simulink model "sampleModel26"  (Simulink 9.1)
settings: Solver=VariableStepAuto  StartTime=0.0  StopTime=10.0  RelTol=1e-3
undefined symbols (not defined in the file): DiscIntNeverNeededParam, Newton, Raphson
libraries: simulink x50
(part 2 of 2)

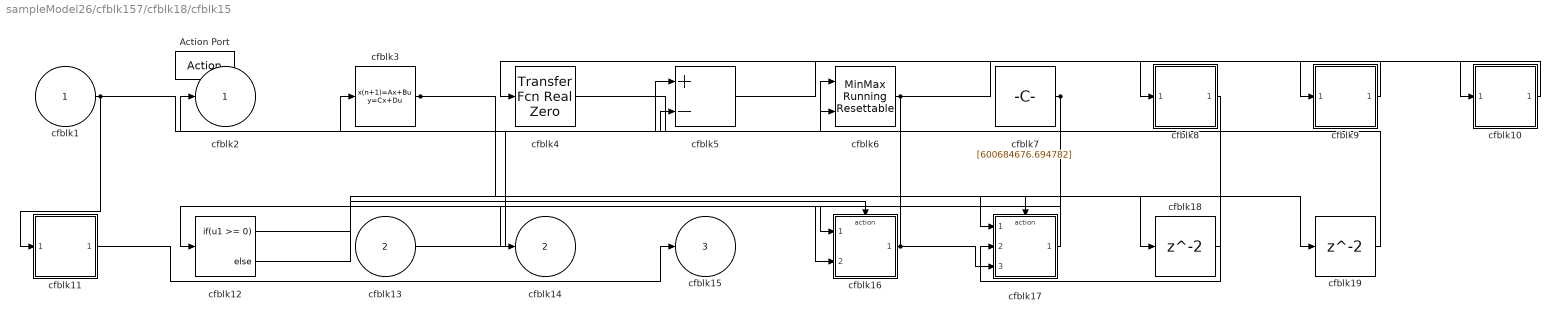
== system sampleModel26/cfblk157/cfblk18/cfblk15 ==
  cfblk1 : Inport
  cfblk13 : Inport  Port=2
  Action Port : ActionPort  ActionType=else
  cfblk10 : Subsystem
  cfblk11 : Subsystem
  cfblk12 : If  IfExpression=u1 >= 0  SampleTime=1
  cfblk16 : Subsystem  TreatAsAtomicUnit=on
  cfblk17 : Subsystem  TreatAsAtomicUnit=on
  cfblk18 : Delay
  cfblk19 : Delay
  cfblk3 : DiscreteStateSpace  SampleTime=-1
  cfblk4 : simulink/Discrete/Transfer Fcn Real Zero  ZeroZ=0.75  ICPrevInput=0.0  DoSatur=off
      settings: SourceProductName=Simulink  SourceProductBaseCode=SL
  cfblk5 : Sum  Inputs=+-
  cfblk6 : simulink/Math Operations/MinMax Running Resettable  Function=min  vinit=0.0
  cfblk7 : Constant  Value=[600684676.694782]  SampleTime=1
  cfblk8 : Subsystem
  cfblk9 : Subsystem
  cfblk2 : Outport
  cfblk14 : Outport  Port=2
  cfblk15 : Outport  Port=3
  wires:
  cfblk10/1(cfblk2) -> cfblk4/1
  cfblk3/1 -> cfblk18/1, cfblk19/1
  cfblk13/1 -> cfblk6/1
  cfblk1/1 -> cfblk11/1(cfblk1), cfblk5/2
  cfblk6/1 -> cfblk12/1, cfblk9/1(cfblk1)
  cfblk4/1 -> cfblk6/2
  cfblk5/1 -> cfblk10/1(cfblk1)
  cfblk11/1(cfblk2) -> cfblk15/1
  cfblk8/1(cfblk2) -> cfblk17/2(cfblk7)
  cfblk7/1 -> cfblk16/1(cfblk1), cfblk16/2(cfblk10), cfblk14/1
  cfblk17/1(cfblk2) -> cfblk2/1
  cfblk9/1(cfblk2) -> cfblk8/1(cfblk1)
  cfblk16/1(cfblk2) -> cfblk17/3(cfblk8), cfblk3/1
  cfblk12/1 -> cfblk16/Action
  cfblk12/2 -> cfblk17/Action
  cfblk18/1 -> cfblk17/1(cfblk1)
  cfblk19/1 -> cfblk5/1

== system sampleModel26/cfblk157/cfblk18/cfblk5 ==
  cfblk1 : Inport
  cfblk2 : Outport
  wires:
  cfblk1/1 -> cfblk2/1

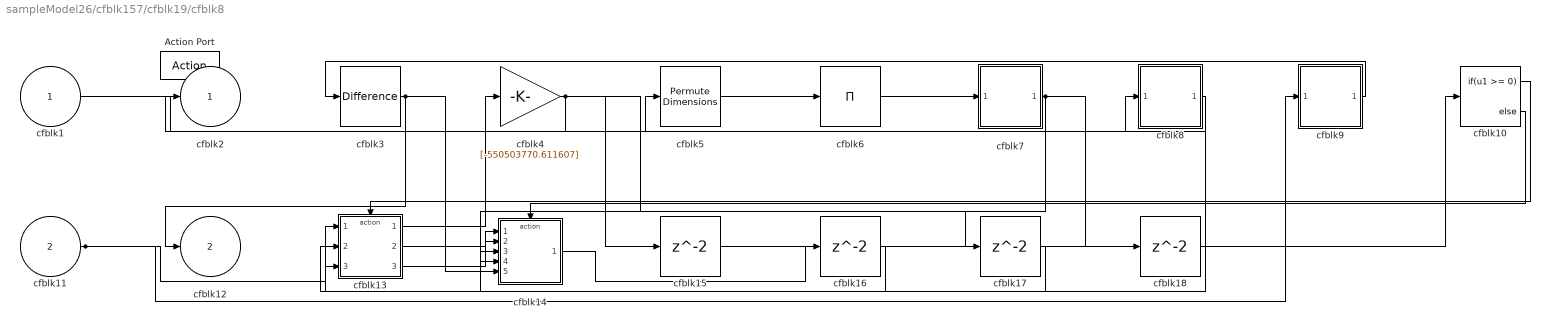
== system sampleModel26/cfblk157/cfblk19/cfblk8 ==
  cfblk1 : Inport
  cfblk11 : Inport  Port=2
  Action Port : ActionPort  ActionType=then
  cfblk10 : If  IfExpression=u1 >= 0  SampleTime=1
  cfblk13 : Subsystem  TreatAsAtomicUnit=on
  cfblk14 : Subsystem  TreatAsAtomicUnit=on
  cfblk{15..18} (4 alike) : Delay
  cfblk3 : simulink/Discrete/Difference  ICPrevInput=0.0  OutMin=[]  OutMax=[]  OutDataTypeStr=Inherit: Inherit via back propagation  OutDataType=fixdt(1, 16)  OutScaling=2^-10  DoSatur=off
  cfblk4 : Gain  Gain=[-550503770.611607]
  cfblk5 : PermuteDimensions
  cfblk6 : Product  Inputs=*
  cfblk7 : Subsystem
  cfblk8 : Subsystem
  cfblk9 : Subsystem
  cfblk2 : Outport
  cfblk12 : Outport  Port=2
  wires:
  cfblk6/1 -> cfblk7/1(cfblk1)
  cfblk1/1 -> cfblk8/1(cfblk1)
  cfblk5/1 -> cfblk6/1
  cfblk9/1(cfblk2) -> cfblk3/1
  cfblk3/1 -> cfblk12/1, cfblk14/5(cfblk17)
  cfblk13/1(cfblk2) -> cfblk4/1
  cfblk4/1 -> cfblk2/1, cfblk15/1, cfblk17/1
  cfblk7/1(cfblk2) -> cfblk14/4(cfblk16), cfblk18/1
  cfblk8/1(cfblk2) -> cfblk13/1(cfblk1)
  cfblk11/1 -> cfblk9/1(cfblk1), cfblk13/3(cfblk14)
  cfblk13/2(cfblk15) -> cfblk14/1(cfblk1)
  cfblk13/3(cfblk16) -> cfblk14/2(cfblk14)
  cfblk10/1 -> cfblk13/Action
  cfblk10/2 -> cfblk14/Action
  cfblk15/1 -> cfblk10/1
  cfblk14/1(cfblk2) -> cfblk16/1
  cfblk16/1 -> cfblk13/2(cfblk13)
  cfblk17/1 -> cfblk14/3(cfblk15)
  cfblk18/1 -> cfblk5/1

== system sampleModel26/cfblk157/cfblk19/cfblk9 ==
  cfblk1 : Inport
  cfblk14 : Inport  Port=2
  cfblk15 : Inport  Port=3
  Action Port : ActionPort  ActionType=else
  cfblk10 : Subsystem
  cfblk11 : Subsystem
  cfblk12 : Subsystem
  cfblk13 : Subsystem
  cfblk3 : simulink/Continuous/PID Controller (2DOF)  Controller=PID  TimeDomain=Discrete-time  SampleTime=-1  IntegratorMethod=Forward Euler  FilterMethod=Forward Euler  Form=Parallel  UseFilter=on  ControllerParametersSource=internal  P=1  I=1  D=0  N=100  b=1  c=1  InitialConditionSource=internal  InitialConditionForIntegrator=0  InitialConditionForFilter=0  ExternalReset=none  LimitOutput=off  UpperSaturationLimit=inf  LowerSaturationLimit=-inf  LinearizeAsGain=off  AntiWindupMode=none  Kb=1  TrackingMode=off  Kt=1  PParamMin=[]  PParamMax=[]  IParamMin=[]  IParamMax=[]  DParamMin=[]  DParamMax=[]  NParamMin=[]  NParamMax=[]  bParamMin=[]  bParamMax=[]  cParamMin=[]  cParamMax=[]  KbParamMin=[]  KbParamMax=[]  KtParamMin=[]  KtParamMax=[]  POutMin=[]  POutMax=[]  IOutMin=[]  IOutMax=[]  DOutMin=[]  DOutMax=[]  NOutMin=[]  NOutMax=[]  bOutMin=[]  bOutMax=[]  cOutMin=[]  cOutMax=[]  KbOutMin=[]  KbOutMax=[]  KtOutMin=[]  KtOutMax=[]  IntegratorOutMin=[]  IntegratorOutMax=[]  FilterOutMin=[]  FilterOutMax=[]  SumOutMin=[]  SumOutMax=[]  Sum1OutMin=[]  Sum1OutMax=[]  Sum2OutMin=[]  Sum2OutMax=[]  Sum3OutMin=[]  Sum3OutMax=[]  SumI1OutMin=[]  SumI1OutMax=[]  SumI2OutMin=[]  SumI2OutMax=[]  SumI3OutMin=[]  SumI3OutMax=[]  SumDOutMin=[]  SumDOutMax=[]  SaturationOutMin=[]  SaturationOutMax=[]  IntegratorContinuousStateAttributes=''  IntegratorStateMustResolveToSignalObject=off  IntegratorRTWStateStorageClass=Auto  FilterContinuousStateAttributes=''  FilterStateMustResolveToSignalObject=off  FilterRTWStateStorageClass=Auto  DifferentiatorICPrevScaledInput=0  DifferentiatorOutMin=[]  DifferentiatorOutMax=[]  FilterDiffOutCoefMin=[]  FilterDiffOutCoefMax=[]  SumDenOutMin=[]  SumDenOutMax=[]  SumNumOutMin=[]  SumNumOutMax=[]  ReciprocalOutMin=[]  ReciprocalOutMax=[]  DivideOutMin=[]  DivideOutMax=[]  TunerSelectOption=Transfer Function Based (PID Tuner App)
  cfblk4 : Sin  TimeSource=Use external signal  SampleTime=0
  cfblk5 : Sqrt  Operator=rSqrt  AlgorithmType=Newton-Raphson  SaturateOnIntegerOverflow=on
  cfblk6 : Sum  Inputs=-+
  cfblk7 : Constant  Value=[532303264.027651]  SampleTime=1
  cfblk8 : Constant  Value=[583399414.909313]  SampleTime=1
  cfblk9 : Subsystem
  cfblk2 : Outport
  cfblk16 : Outport  Port=2
  wires:
  cfblk6/1 -> cfblk10/1(cfblk1)
  cfblk11/1(cfblk2) -> cfblk4/1
  cfblk3/1 -> cfblk9/1(cfblk1)
  cfblk12/1(cfblk2) -> cfblk2/1
  cfblk13/1(cfblk2) -> cfblk5/1
  cfblk10/1(cfblk2) -> cfblk12/1(cfblk1)
  cfblk8/1 -> cfblk13/1(cfblk1)
  cfblk5/1 -> cfblk6/1
  cfblk9/1(cfblk2) -> cfblk16/1
  cfblk7/1 -> cfblk3/1
  cfblk4/1 -> cfblk6/2
  cfblk14/1 -> cfblk3/2
  cfblk15/1 -> cfblk11/1(cfblk1)

== system sampleModel26/cfblk160/cfblk17/cfblk11 ==
  cfblk1 : Inport
  cfblk2 : Outport
  wires:
  cfblk1/1 -> cfblk2/1

== system sampleModel26/cfblk160/cfblk18/cfblk6 ==
  cfblk1 : Inport
  cfblk2 : Outport
  wires:
  cfblk1/1 -> cfblk2/1

== system sampleModel26/cfblk160/cfblk18/cfblk7 ==
  cfblk1 : Inport
  cfblk2 : Outport
  wires:
  cfblk1/1 -> cfblk2/1

== system sampleModel26/cfblk160/cfblk18/cfblk8 ==
  cfblk1 : Inport
  cfblk2 : Outport
  wires:
  cfblk1/1 -> cfblk2/1

== system sampleModel26/cfblk160/cfblk18/cfblk9 ==
  cfblk1 : Inport
  cfblk2 : Outport
  wires:
  cfblk1/1 -> cfblk2/1

== system sampleModel26/cfblk157/cfblk18/cfblk12/cfblk13 ==
  cfblk1 : Inport
  cfblk12 : Inport  Port=2
  cfblk13 : Inport  Port=3
  Action Port : ActionPort  ActionType=then
  cfblk10 : Sum  Inputs=+-
  cfblk11 : Constant  Value=[603434454.897052]  SampleTime=1
  cfblk3 : DiscreteFir
  cfblk4 : DiscreteTransferFcn
  cfblk5 : DiscreteTransferFcn
  cfblk6 : Delay
  cfblk7 : simulink/Discrete/Transfer Fcn First Order  PoleZ=0.95  ICPrevOutput=0.0  DoSatur=off
      settings: SourceProductName=Simulink
  cfblk8 : Rounding
  cfblk9 : PermuteDimensions
  cfblk2 : Outport
  wires:
  cfblk6/1 -> cfblk8/1
  cfblk12/1 -> cfblk7/1
  cfblk1/1 -> cfblk2/1
  cfblk11/1 -> cfblk9/1
  cfblk9/1 -> cfblk4/1
  cfblk4/1 -> cfblk6/1
  cfblk7/1 -> cfblk5/1
  cfblk13/1 -> cfblk3/1
  cfblk3/1 -> cfblk10/1
  cfblk5/1 -> cfblk10/2

== system sampleModel26/cfblk157/cfblk18/cfblk12/cfblk14 ==
  cfblk1 : Inport
  cfblk14 : Inport  Port=2
  cfblk15 : Inport  Port=3
  Action Port : ActionPort  ActionType=else
  cfblk10 : Sum  Inputs=|++
  cfblk11 : Sum  Inputs=+-
  cfblk12 : simulink/Math Operations/Slider Gain  gain=1  low=0  high=2
  cfblk13 : Constant  Value=[170798699.836633]  SampleTime=1
  cfblk3 : simulink/Discrete/Transfer Fcn First Order  PoleZ=0.95  ICPrevOutput=0.0  DoSatur=off
      settings: SourceProductName=Simulink
  cfblk4 : DiscreteZeroPole  Poles=[0 0.5]  Gain=1  SampleTime=-1
  cfblk5 : Delay
  cfblk6 : DiscreteTransferFcn
  cfblk7 : Sqrt  Operator=rSqrt  AlgorithmType=Newton-Raphson  SaturateOnIntegerOverflow=on
  cfblk8 : Polyval  Coefs=[ +2.081618890e-019, -1.441693666e-014, +4.719686976e-010, -8.536869453e-006, +1.621573104e-001, -8.087801117e+001 ]
  cfblk9 : Sin  TimeSource=Use external signal  SampleTime=0
  cfblk2 : Outport
  cfblk16 : Outport  Port=2
  wires:
  cfblk5/1 -> cfblk4/1
  cfblk14/1 -> cfblk10/1
  cfblk13/1 -> cfblk5/1
  cfblk10/1 -> cfblk3/1
  cfblk11/1 -> cfblk16/1
  cfblk7/1 -> cfblk9/1
  cfblk8/1 -> cfblk2/1
  cfblk4/1 -> cfblk7/1
  cfblk6/1 -> cfblk11/1
  cfblk1/1 -> cfblk12/1
  cfblk9/1 -> cfblk11/2
  cfblk12/1 -> cfblk10/2
  cfblk15/1 -> cfblk6/1
  cfblk3/1 -> cfblk8/1

== system sampleModel26/cfblk157/cfblk18/cfblk12/cfblk9 ==
  cfblk1 : Inport
  cfblk2 : Outport
  wires:
  cfblk1/1 -> cfblk2/1

== system sampleModel26/cfblk157/cfblk18/cfblk13/cfblk8 ==
  cfblk1 : Inport
  cfblk2 : Outport
  wires:
  cfblk1/1 -> cfblk2/1

== system sampleModel26/cfblk157/cfblk18/cfblk14/cfblk4 ==
  cfblk1 : Inport
  cfblk2 : Outport
  wires:
  cfblk1/1 -> cfblk2/1

== system sampleModel26/cfblk157/cfblk18/cfblk14/cfblk5 ==
  cfblk1 : Inport
  cfblk2 : Outport
  wires:
  cfblk1/1 -> cfblk2/1

== system sampleModel26/cfblk157/cfblk18/cfblk14/cfblk6 ==
  cfblk1 : Inport
  cfblk2 : Outport
  wires:
  cfblk1/1 -> cfblk2/1

== system sampleModel26/cfblk157/cfblk18/cfblk15/cfblk10 ==
  cfblk1 : Inport
  cfblk2 : Outport
  wires:
  cfblk1/1 -> cfblk2/1

== system sampleModel26/cfblk157/cfblk18/cfblk15/cfblk11 ==
  cfblk1 : Inport
  cfblk2 : Outport
  wires:
  cfblk1/1 -> cfblk2/1

== system sampleModel26/cfblk157/cfblk18/cfblk15/cfblk16 ==
  cfblk1 : Inport
  cfblk10 : Inport  Port=2
  Action Port : ActionPort  ActionType=then
  cfblk11 : Delay
  cfblk12 : Delay
  cfblk3 : UnitDelay  SampleTime=-1
  cfblk4 : simulink/Continuous/PID Controller (2DOF)  Controller=PID  TimeDomain=Discrete-time  SampleTime=-1  IntegratorMethod=Forward Euler  FilterMethod=Forward Euler  Form=Parallel  UseFilter=on  ControllerParametersSource=internal  P=1  I=1  D=0  N=100  b=1  c=1  InitialConditionSource=internal  InitialConditionForIntegrator=0  InitialConditionForFilter=0  ExternalReset=none  LimitOutput=off  UpperSaturationLimit=inf  LowerSaturationLimit=-inf  LinearizeAsGain=off  AntiWindupMode=none  Kb=1  TrackingMode=off  Kt=1  PParamMin=[]  PParamMax=[]  IParamMin=[]  IParamMax=[]  DParamMin=[]  DParamMax=[]  NParamMin=[]  NParamMax=[]  bParamMin=[]  bParamMax=[]  cParamMin=[]  cParamMax=[]  KbParamMin=[]  KbParamMax=[]  KtParamMin=[]  KtParamMax=[]  POutMin=[]  POutMax=[]  IOutMin=[]  IOutMax=[]  DOutMin=[]  DOutMax=[]  NOutMin=[]  NOutMax=[]  bOutMin=[]  bOutMax=[]  cOutMin=[]  cOutMax=[]  KbOutMin=[]  KbOutMax=[]  KtOutMin=[]  KtOutMax=[]  IntegratorOutMin=[]  IntegratorOutMax=[]  FilterOutMin=[]  FilterOutMax=[]  SumOutMin=[]  SumOutMax=[]  Sum1OutMin=[]  Sum1OutMax=[]  Sum2OutMin=[]  Sum2OutMax=[]  Sum3OutMin=[]  Sum3OutMax=[]  SumI1OutMin=[]  SumI1OutMax=[]  SumI2OutMin=[]  SumI2OutMax=[]  SumI3OutMin=[]  SumI3OutMax=[]  SumDOutMin=[]  SumDOutMax=[]  SaturationOutMin=[]  SaturationOutMax=[]  IntegratorContinuousStateAttributes=''  IntegratorStateMustResolveToSignalObject=off  IntegratorRTWStateStorageClass=Auto  FilterContinuousStateAttributes=''  FilterStateMustResolveToSignalObject=off  FilterRTWStateStorageClass=Auto  DifferentiatorICPrevScaledInput=0  DifferentiatorOutMin=[]  DifferentiatorOutMax=[]  FilterDiffOutCoefMin=[]  FilterDiffOutCoefMax=[]  SumDenOutMin=[]  SumDenOutMax=[]  SumNumOutMin=[]  SumNumOutMax=[]  ReciprocalOutMin=[]  ReciprocalOutMax=[]  DivideOutMin=[]  DivideOutMax=[]  TunerSelectOption=Transfer Function Based (PID Tuner App)
  cfblk5 : Sqrt  SaturateOnIntegerOverflow=on
  cfblk6 : simulink/Math Operations/MinMax Running Resettable  Function=min  vinit=0.0
  cfblk7 : ComplexToRealImag
  cfblk8 : Sum  Inputs=+
  cfblk9 : Constant  Value=[-275406093.401909]  SampleTime=1
  cfblk2 : Outport
  wires:
  cfblk6/1 -> cfblk5/1
  cfblk4/1 -> cfblk8/1
  cfblk5/1 -> cfblk3/1
  cfblk3/1 -> cfblk7/1
  cfblk10/1 -> cfblk2/1
  cfblk1/1 -> cfblk4/2
  cfblk8/1 -> cfblk6/2
  cfblk7/1 -> cfblk11/1
  cfblk11/1 -> cfblk4/1
  cfblk7/2 -> cfblk12/1
  cfblk12/1 -> cfblk6/1

== system sampleModel26/cfblk157/cfblk18/cfblk15/cfblk17 ==
  cfblk1 : Inport
  cfblk7 : Inport  Port=2
  cfblk8 : Inport  Port=3
  Action Port : ActionPort  ActionType=else
  cfblk3 : Reshape
  cfblk4 : Product  Inputs=**
  cfblk5 : PermuteDimensions
  cfblk6 : ComplexToRealImag
  cfblk2 : Outport
  wires:
  cfblk6/1 -> cfblk2/1
  cfblk1/1 -> cfblk5/1
  cfblk8/1 -> cfblk3/1
  cfblk6/2 -> cfblk4/1
  cfblk5/1 -> cfblk4/2
  cfblk3/1 -> cfblk6/1

== system sampleModel26/cfblk157/cfblk18/cfblk15/cfblk8 ==
  cfblk1 : Inport
  cfblk2 : Outport
  wires:
  cfblk1/1 -> cfblk2/1

== system sampleModel26/cfblk157/cfblk18/cfblk15/cfblk9 ==
  cfblk1 : Inport
  cfblk2 : Outport
  wires:
  cfblk1/1 -> cfblk2/1

== system sampleModel26/cfblk157/cfblk19/cfblk8/cfblk13 ==
  cfblk1 : Inport
  cfblk13 : Inport  Port=2
  cfblk14 : Inport  Port=3
  Action Port : ActionPort  ActionType=then
  cfblk10 : MinMax  Function=max  Inputs=3
  cfblk11 : Constant  Value=[-226330828.269443]  SampleTime=1
  cfblk12 : Constant  Value=[-386479212.114649]  SampleTime=1
  cfblk3 : DiscreteIntegrator  SampleTime=-1  ICPrevOutput=DiscIntNeverNeededParam  ICPrevScaledInput=DiscIntNeverNeededParam
  cfblk4 : DiscreteIntegrator  SampleTime=-1  ICPrevOutput=DiscIntNeverNeededParam  ICPrevScaledInput=DiscIntNeverNeededParam
  cfblk5 : DiscreteFir
  cfblk6 : simulink/Discrete/Transfer Fcn First Order  PoleZ=0.95  ICPrevOutput=0.0  DoSatur=off
      settings: SourceProductName=Simulink
  cfblk7 : simulink/Math Operations/Slider Gain  gain=1  low=0  high=2
  cfblk8 : Gain  Gain=[-242677494.335808]
  cfblk9 : Polyval  Coefs=[ +2.081618890e-019, -1.441693666e-014, +4.719686976e-010, -8.536869453e-006, +1.621573104e-001, -8.087801117e+001 ]
  cfblk2 : Outport
  cfblk15 : Outport  Port=2
  cfblk16 : Outport  Port=3
  wires:
  cfblk11/1 -> cfblk3/1
  cfblk6/1 -> cfblk8/1
  cfblk1/1 -> cfblk7/1
  cfblk10/1 -> cfblk9/1
  cfblk4/1 -> cfblk5/1
  cfblk3/1 -> cfblk6/1
  cfblk5/1 -> cfblk2/1
  cfblk13/1 -> cfblk15/1
  cfblk12/1 -> cfblk4/1
  cfblk9/1 -> cfblk16/1
  cfblk7/1 -> cfblk10/1
  cfblk8/1 -> cfblk10/2
  cfblk14/1 -> cfblk10/3

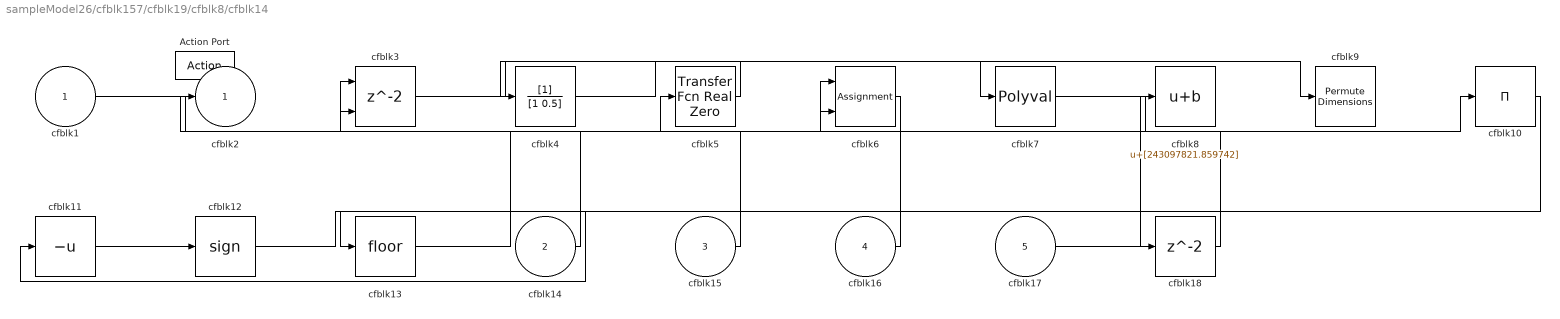
== system sampleModel26/cfblk157/cfblk19/cfblk8/cfblk14 ==
  cfblk1 : Inport
  cfblk14 : Inport  Port=2
  cfblk15 : Inport  Port=3
  cfblk16 : Inport  Port=4
  cfblk17 : Inport  Port=5
  Action Port : ActionPort  ActionType=else
  cfblk10 : Product  Inputs=*
  cfblk11 : UnaryMinus
  cfblk12 : Signum
  cfblk13 : Rounding
  cfblk18 : Delay
  cfblk3 : Delay  ShowEnablePort=on
      settings: InputPortMap=u0,e6
  cfblk4 : DiscreteFilter
  cfblk5 : simulink/Discrete/Transfer Fcn Real Zero  ZeroZ=0.75  ICPrevInput=0.0  DoSatur=off
      settings: SourceProductName=Simulink  SourceProductBaseCode=SL
  cfblk6 : Assignment  DiagnosticForDimensions=Warning  IndexOptions=Index vector (dialog)  Indices=1  OutputSizes=1
  cfblk7 : Polyval  Coefs=[ +2.081618890e-019, -1.441693666e-014, +4.719686976e-010, -8.536869453e-006, +1.621573104e-001, -8.087801117e+001 ]
  cfblk8 : Bias  Bias=[243097821.859742]
  cfblk9 : PermuteDimensions
  cfblk2 : Outport
  wires:
  cfblk14/1 -> cfblk3/1
  cfblk11/1 -> cfblk12/1
  cfblk3/1 -> cfblk9/1
  cfblk1/1 -> cfblk5/1
  cfblk6/1 -> cfblk11/1
  cfblk5/1 -> cfblk4/1
  cfblk7/1 -> cfblk10/1
  cfblk17/1 -> cfblk8/1
  cfblk15/1 -> cfblk3/2
  cfblk16/1 -> cfblk2/1
  cfblk4/1 -> cfblk7/1
  cfblk10/1 -> cfblk13/1
  cfblk13/1 -> cfblk6/1
  cfblk12/1 -> cfblk18/1
  cfblk18/1 -> cfblk6/2

== system sampleModel26/cfblk157/cfblk19/cfblk8/cfblk7 ==
  cfblk1 : Inport
  cfblk2 : Outport
  wires:
  cfblk1/1 -> cfblk2/1

== system sampleModel26/cfblk157/cfblk19/cfblk8/cfblk8 ==
  cfblk1 : Inport
  cfblk2 : Outport
  wires:
  cfblk1/1 -> cfblk2/1

== system sampleModel26/cfblk157/cfblk19/cfblk8/cfblk9 ==
  cfblk1 : Inport
  cfblk2 : Outport
  wires:
  cfblk1/1 -> cfblk2/1

== system sampleModel26/cfblk157/cfblk19/cfblk9/cfblk10 ==
  cfblk1 : Inport
  cfblk2 : Outport
  wires:
  cfblk1/1 -> cfblk2/1

== system sampleModel26/cfblk157/cfblk19/cfblk9/cfblk11 ==
  cfblk1 : Inport
  cfblk2 : Outport
  wires:
  cfblk1/1 -> cfblk2/1

== system sampleModel26/cfblk157/cfblk19/cfblk9/cfblk12 ==
  cfblk1 : Inport
  cfblk2 : Outport
  wires:
  cfblk1/1 -> cfblk2/1

== system sampleModel26/cfblk157/cfblk19/cfblk9/cfblk13 ==
  cfblk1 : Inport
  cfblk2 : Outport
  wires:
  cfblk1/1 -> cfblk2/1

== system sampleModel26/cfblk157/cfblk19/cfblk9/cfblk9 ==
  cfblk1 : Inport
  cfblk2 : Outport
  wires:
  cfblk1/1 -> cfblk2/1
